simulink model "biogas"  (R2020a)
settings: Solver=VariableStepAuto  StartTime=0.0  StopTime=50  RelTol=1e-3
libraries: simulink x1
settings Model: Creator=Reaga  LastModifiedBy=Reaga

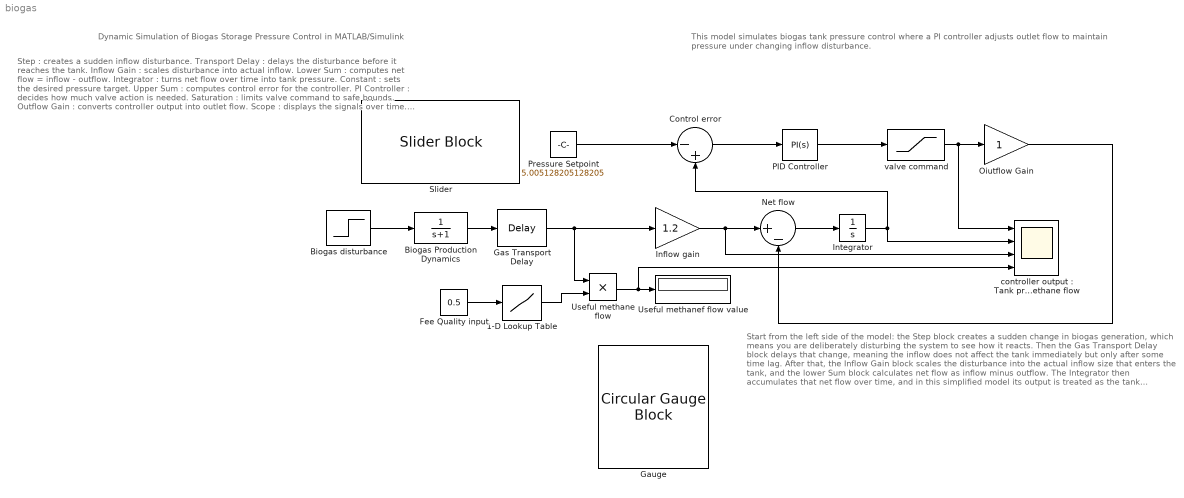
== system biogas ==
  note: Start from the left side of the model: the Step block creates a sudden change in biogas generation, which means you are deliberately disturbing the system to see how it reacts. Then the Gas Transport Delay block delays that change, meaning the inflow does not affect the tank immediately but only after some time lag.
      | After that, the Inflow Gain block scales the disturbance into the actual inflow size that enters the tank, and the lower Sum block calculates net flow as inflow minus outflow. The Integrator then accumulates that net flow over time, and in this simplified model its output is treated as the tank pressure .
      | At the top, the Constant block gives the desired pressure setpoint, and the upper Sum block creates the control error, which is the signal telling the controller how far the system is from the target. The PI controller takes that error and creates a control action, meaning it decides how much the outlet valve should respond to bring pressure back toward the setpoint.
      | The Saturation block limits that controller output so the valve command stays within a realistic range, and the Outflow Gain turns that valve command into the outflow leaving the tank. That outflow goes back to the lower Sum block, so if the controller increases outflow, the tank pressure stops rising as much or starts dropping, which is how the system regulates itself.
      | the bottom plot is the delayed inflow disturbance, so it shows when the inflow changes and how the transport delay shifts that change to a later time. The middle plot is the tank pressure, so this is the main result showing how pressure rises, overshoots a bit, and then settles back near the target value. The top plot is the controller output or valve command, which shows how strongly the controller reacts when the disturbance happens or when the setpoint changes.
      | If you change the Feed Quality input constant, the output of the lookup table will also change, because a lookup table maps input values to output values based on the breakpoints and table data you entered.
  note: This model simulates biogas tank pressure control where a PI controller adjusts outlet flow to maintain pressure under changing inflow disturbance.
  note: Step : creates a sudden inflow disturbance.
      | Transport Delay : delays the disturbance before it reaches the tank.
      | Inflow Gain : scales disturbance into actual inflow.
      | Lower Sum : computes net flow = inflow - outflow.
      | Integrator : turns net flow over time into tank pressure.
      | Constant : sets the desired pressure target.
      | Upper Sum : computes control error for the controller.
      | PI Controller : decides how much valve action is needed.
      | Saturation : limits valve command to safe bounds.
      | Outflow Gain : converts controller output into outlet flow.
      | Scope : displays the signals over time.
      | Slider : changes the setpoint interactively during simulation.
      | Biogas Production Dynamics — Represents the gradual response of biogas generation to a change in biomass feed instead of an instantaneous change.
      | Useful methane flow — Calculates the methane-rich usable portion of the delayed biogas flow by multiplying total biogas flow by methane fraction.
      | biogas comes in, the tank pressure changes, and a PI controller opens or closes the outlet valve to keep the pressure near the target value you set. It is not a full biochemical digestion model; it is a simplified control-system model made to show disturbance, delay, feedback, and tuning in Simulink.The setpoint is just the pressure you want, the actual pressure is what the tank currently has, and the controller uses the difference between them to decide what to do next.
  note: Dynamic Simulation of Biogas Storage Pressure Control in MATLAB/Simulink
  1-D Lookup Table : Lookup_n-D  NumberOfTableDimensions=1  BreakpointsForDimension1=[0.8 0.9 1.0]  Table=[0.50 0.60 0.70]  InternalRulePriority=Speed  RndMeth=Simplest  InputSameDT=on
  Biogas disturbance : Step  Time=10  Before=0.5  SampleTime=0
  Biogas Production Dynamics : TransferFcn  Denominator=[1 1]
  Control error : Sum  Inputs=|-+
  Fee Quality input : Constant  Value=0.5
  Gas Transport Delay : TransportDelay  DelayTime=2
  Gauge : CircularGaugeBlock  ScaleMax=1
  Inflow gain : Gain  Gain=1.2
  Integrator : Integrator  InitialCondition=4.5
  Net flow : Sum  Inputs=|+-
  Oiutflow Gain : Gain
  PID Controller : simulink/Continuous/PID Controller  Controller=PI  Form=Parallel  TimeDomain=Continuous-time  UseExternalTs=off  SampleTime=-1  IntegratorMethod=Forward Euler  FilterMethod=Forward Euler  ControllerParametersSource=internal  P=2  I=0.8  D=0  UseFilter=on  N=100  TunerSelectOption=Transfer Function Based (PID Tuner App)  InitialConditionSource=internal  InitialConditionForIntegrator=0  InitialConditionForFilter=0  DifferentiatorICPrevScaledInput=0  ExternalReset=none  TrackingMode=off  Kt=1  LimitOutput=off  UpperSaturationLimit=inf  LowerSaturationLimit=-inf  LinearizeAsGain=on  AntiWindupMode=none  Kb=1  POutMin=[]  POutMax=[]  IOutMin=[]  IOutMax=[]  DOutMin=[]  DOutMax=[]  NOutMin=[]  NOutMax=[]  SumOutMin=[]  SumOutMax=[]  SaturationOutMin=[]  SaturationOutMax=[]  PParamMin=[]  PParamMax=[]  IParamMin=[]  IParamMax=[]  DParamMin=[]  DParamMax=[]  NParamMin=[]  NParamMax=[]  KbParamMin=[]  KbParamMax=[]  KtParamMin=[]  KtParamMax=[]  KbOutMin=[]  KbOutMax=[]  KtOutMin=[]  KtOutMax=[]  IntegratorOutMin=[]  IntegratorOutMax=[]  FilterOutMin=[]  FilterOutMax=[]  SumI1OutMin=[]  SumI1OutMax=[]  SumI2OutMin=[]  SumI2OutMax=[]  SumI3OutMin=[]  SumI3OutMax=[]  SumI4OutMin=[]  SumI4OutMax=[]  SumDOutMin=[]  SumDOutMax=[]  DifferentiatorOutMin=[]  DifferentiatorOutMax=[]  FilterDiffOutCoefMin=[]  FilterDiffOutCoefMax=[]  ReciprocalOutMin=[]  ReciprocalOutMax=[]  SumDenOutMin=[]  SumDenOutMax=[]  SumNumOutMin=[]  SumNumOutMax=[]  DivideOutMin=[]  DivideOutMax=[]  UdiffTsProdOutMin=[]  UdiffTsProdOutMax=[]  NTsProdOutMin=[]  NTsProdOutMax=[]  UintegralTsProdOutMin=[]  UintegralTsProdOutMax=[]  UngainTsProdOutMin=[]  UngainTsProdOutMax=[]  IntegratorContinuousStateAttributes=''  IntegratorStateMustResolveToSignalObject=off  IntegratorRTWStateStorageClass=Auto  FilterContinuousStateAttributes=''  FilterStateMustResolveToSignalObject=off  FilterRTWStateStorageClass=Auto  ParallelPVariant=InternalParameters  IdealPVariant=Disabled  IVariant=InternalParameters  DVariant=Disabled  IntegratorVariant=Continuous  SatVariant=Disabled  AWVariant=Passthrough  PCopyVariant=Disabled  TRVariant=Disabled  FdbkBlocksVariant=Forward  IdealPFdbkVariant=Disabled  SatFdbkVariant=Disabled  DerivativeFilterVariant=Disabled  NVariant=Disabled  NCopyVariant=Disabled_SignalSpec  FilterICVariant=Disabled  IntegratorICVariant=InternalICs  ExternalResetVariant=Disabled  TRSumVariant=Passthrough  SumFdbkVariant=Disabled  SumVariant=Sum_PI  TsampFilterVariant=InternalTs  TsampNgainVariant=Passthrough  TsampIntegralVariant=Passthrough
  Pressure Setpoint : Constant  Value=5.005128205128205
  Slider : SliderBlock  ScaleMin=4  ScaleMax=6  TickInterval=0.5
  Useful methane flow : Product
  Useful methanef flow value : Display
  "controller output : Tank pressure : Delayed biogas inflow : Useful methane flow" : Scope  NumInputPorts=4
  valve command : Saturate  UpperLimit=2  LowerLimit=0
  wires:
  Integrator/1 -> "controller output : Tank pressure : Delayed biogas inflow : Useful methane flow"/2, Control error/2
  Inflow gain/1 -> Net flow/1, "controller output : Tank pressure : Delayed biogas inflow : Useful methane flow"/3
  Net flow/1 -> Integrator/1
  Pressure Setpoint/1 -> Control error/1
  Control error/1 -> PID Controller/1
  PID Controller/1 -> valve command/1
  valve command/1 -> "controller output : Tank pressure : Delayed biogas inflow : Useful methane flow"/1, Oiutflow Gain/1
  Oiutflow Gain/1 -> Net flow/2
  Biogas disturbance/1 -> Biogas Production Dynamics/1
  Biogas Production Dynamics/1 -> Gas Transport Delay/1
  Gas Transport Delay/1 -> Useful methane flow/1, Inflow gain/1
  Useful methane flow/1 -> "controller output : Tank pressure : Delayed biogas inflow : Useful methane flow"/4, Useful methanef flow value/1
  Fee Quality input/1 -> 1-D Lookup Table/1
  1-D Lookup Table/1 -> Useful methane flow/2
